simulink model "triangle"  (R2018b)
settings: Solver=FixedStepAuto  StartTime=0.0  StopTime=inf  FixedStep=1/20  RelTol=1e-3  EnableMultiTasking=on
PreLoadFcn:
  | triangle_startup
settings Model: SimulationMode=external  Creator=Josef  LastModifiedBy=Josef
settings SolverCC: PositivePriorityOrder=on
settings OptimizationCC: PassReuseOutputArgsThreshold=0  MaxStackSize=64
settings DebuggingCC: ParameterTunabilityLossMsg=error
settings HardwareCC: ProdBitPerPointer=32  ProdBitPerSizeT=32  ProdBitPerPtrDiffT=32  ProdLargestAtomicInteger=Long  ProdLargestAtomicFloat=Double  ProdWordSize=32  ProdHWDeviceType=ARM Compatible->ARM Cortex  UseEmbeddedCoderFeatures=off
settings SFSimCC: SimUseLocalCustomCode=off  MATLABDynamicMemAlloc=off
settings RTWCC: SystemTargetFile=ert.tlc  HardwareBoard=Raspberry Pi  TLCOptions="-aInlineSetEventsForThisBaseRateFcn=TLC_FALSE -aSuppressMultiTaskScheduler=TLC_FALSE  -aRateBasedStepFcn=0"  TemplateMakefile=ert_default_tmf  GenerateReport=on  RTWUseLocalCustomCode=off  Toolchain=GNU GCC Raspberry Pi  TargetLang=C++
settings CodeAppCC: ForceParamTrailComments=on  OperatorAnnotations=on
settings ERTTargetCC: TargetLangStandard=C++03 (ISO)  ERTCustomFileBanners=off  SupportContinuousTime=on  SupportNonInlinedSFcns=on  RemoveResetFunc=off  SupportVariableSizeSignals=on  ModelStepFunctionPrototypeControlCompliant=off

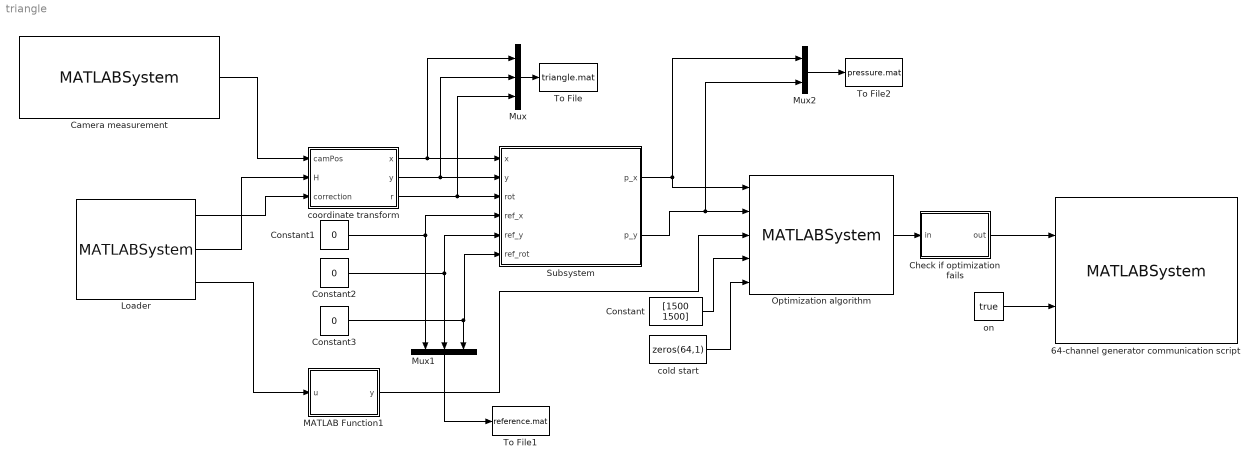
== system triangle ==
  64-channel generator communication script : MATLABSystem  System=NewGenerator  Port=/dev/ttyUSB0  Baud=230400
      mask Type: NewGenerator
      mask Display:
      | disp(['64 phase generator' char(10) ' Port: /dev/ttyUSB0' char(10) ' Baudrate: 230400']);
      | port_label('input',1,'phases');
      | port_label('input',2,'On/Off');
  Camera measurement : MATLABSystem  System=RaspiBallPos  shm_key=3145914  framerate=50  N=1000  objects=1  km=eye( 3 )  notfound=0  execScript=off  concatenateOutputs=off  rotation=on  found_output=off
      mask Type: RaspiBallPos
      mask Display:
      | disp('RaspiBallPos');
      | port_label('output',1,'Position 1 [x;y;r]');
  Check if optimization fails : MATLAB Function  TreatAsAtomicUnit=on
  Constant : Constant  Value=[1500 1500]
  Constant1 : Constant  Value=0
  Constant2 : Constant  Value=0
  Constant3 : Constant  Value=0
  Loader : MATLABSystem  System=Loader  corrFile=correction.bin  H_unFile=H_unrot.bin  heightFile=height.bin
      mask Type: Loader
      mask Display:
      | disp('Loader');
      | port_label('output',1,'correction');
      | port_label('output',2,'H_unrot');
      | port_label('output',3,'height');
  MATLAB Function1 : MATLAB Function  TreatAsAtomicUnit=on
  Mux : Mux  Inputs=3
  Mux1 : Mux  Inputs=3
  Mux2 : Mux  Inputs=2
  Optimization algorithm : MATLABSystem  System=PressurePoints
      mask Type: PressurePoints
      mask Display:
      | disp(['Pressure points' char(10) 'optimization']);
      | port_label('input',1,'x');
      | port_label('input',2,'y');
      | port_label('input',3,'z');
      | port_label('input',4,'Required pressure');
      | port_label('input',5,'Initial condition');
      | port_label('output',1,'Phases');
  Subsystem : Subsystem  mask{triangle_width=0.010, triangle_height=0.013, in_dist=0.0015, out_dist=0.00075}
      mask prompts: triangle_width "Width"; triangle_height "Height"; in_dist "Inner distance"; out_dist "Outer distance"
      mask DialogControl DescGroupVar Prompt: Controller
      mask DialogControl DescTextVar Prompt: Determines position of high-pressure points
      mask DialogControl Container3 Prompt: Triangle
      mask DialogControl Container4 Prompt: Determine pressure points
  To File : ToFile  Filename=triangle.mat  MatrixName=triangle
  To File1 : ToFile  Filename=reference.mat  MatrixName=reference
  To File2 : ToFile  Filename=pressure.mat  MatrixName=pressure
  cold start : Constant  Value=zeros(64,1)
  coordinate transform : MATLAB Function  TreatAsAtomicUnit=on
  on : Constant  Value=true
  wires:
  Camera measurement/1 -> coordinate transform/1(camPos)
  Optimization algorithm/1 -> Check if optimization fails/1(in)
  cold start/1 -> Optimization algorithm/5
  on/1 -> 64-channel generator communication script/2
  Check if optimization fails/1(out) -> 64-channel generator communication script/1
  Loader/1 -> coordinate transform/3(correction)
  Loader/2 -> coordinate transform/2(H)
  Loader/3 -> MATLAB Function1/1(u)
  MATLAB Function1/1(y) -> Optimization algorithm/3
  Constant/1 -> Optimization algorithm/4
  coordinate transform/1(x) -> Mux/1, Subsystem/1(x)
  coordinate transform/2(y) -> Mux/2, Subsystem/2(y)
  coordinate transform/3(r) -> Mux/3, Subsystem/3(rot)
  Constant1/1 -> Subsystem/4(ref_x), Mux1/1
  Constant2/1 -> Subsystem/5(ref_y), Mux1/2
  Constant3/1 -> Subsystem/6(ref_rot), Mux1/3
  Subsystem/1(p_x) -> Mux2/1, Optimization algorithm/1
  Subsystem/2(p_y) -> Mux2/2, Optimization algorithm/2
  Mux/1 -> To File/1
  Mux1/1 -> To File1/1
  Mux2/1 -> To File2/1

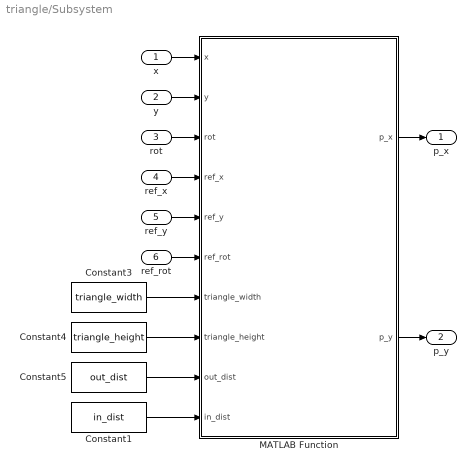
== system triangle/Subsystem ==
  x : Inport
  y : Inport  Port=2
  rot : Inport  Port=3
  ref_x : Inport  Port=4
  ref_y : Inport  Port=5
  ref_rot : Inport  Port=6
  Constant1 : Constant  Value=in_dist
  Constant3 : Constant  Value=triangle_width
  Constant4 : Constant  Value=triangle_height
  Constant5 : Constant  Value=out_dist
  MATLAB Function : MATLAB Function  TreatAsAtomicUnit=on
  p_x : Outport
  p_y : Outport  Port=2
  wires:
  MATLAB Function/1(p_x) -> p_x/1
  rot/1 -> MATLAB Function/3(rot)
  Constant3/1 -> MATLAB Function/7(triangle_width)
  x/1 -> MATLAB Function/1(x)
  ref_x/1 -> MATLAB Function/4(ref_x)
  Constant4/1 -> MATLAB Function/8(triangle_height)
  y/1 -> MATLAB Function/2(y)
  Constant5/1 -> MATLAB Function/9(out_dist)
  ref_y/1 -> MATLAB Function/5(ref_y)
  ref_rot/1 -> MATLAB Function/6(ref_rot)
  MATLAB Function/2(p_y) -> p_y/1
  Constant1/1 -> MATLAB Function/10(in_dist)

== matlab function triangle/coordinate transform ==
  data: x output; camPos input; y output; H input; correction input; r output
function [x,y,r] = trans(camPos, H, correction)
    [x,y] = coordTransform(H, camPos(1:2), correction);
    r = camPos(3);
end

== matlab function triangle/Subsystem/MATLAB Function ==
  data: x input; p_x output; y input; rot input; ref_x input; ref_y input; ref_rot input; triangle_width input; triangle_height input; p_y output; out_dist input; in_dist input
function [p_x, p_y] = determine_pressure_points(x, y, rot, ref_x, ref_y, ref_rot, triangle_width, triangle_height, out_dist, in_dist)
    rot_mat = [cos(rot), -sin(rot); sin(rot), cos(rot)];
    ref_rot_mat = [cos(ref_rot), -sin(ref_rot); sin(ref_rot), cos(ref_rot)];
    T = [x;y];
    P = [ref_x;ref_y];
    
    dx = triangle_height/3 + out_dist;
    dy = triangle_width/2 + out_dist;   
    dxr = triangle_height/3 - in_dist;
    dyr = triangle_width/2 - in_dist;
    TA = rot_mat * [-dxr;dyr];
    TB = rot_mat * [-dxr;-dyr];
    TC = rot_mat * [2*dxr;0];
    TP = P - T;
    A = T + TA;
    B = T + TB;
    C = T + TC;
    
    total_dist = in_dist + out_dist;
	AA_ref = - TA + TP + ref_rot_mat * [-dx;dy];
    if norm(AA_ref) > total_dist
        AA_ref = AA_ref / norm(AA_ref) * (total_dist);
    end
	BB_ref = - TB + TP +  ref_rot_mat * [-dx;-dy];
    if norm(BB_ref) > total_dist
        BB_ref = BB_ref / norm(BB_ref) * (total_dist);
    end
	CC_ref = - TC + TP +  ref_rot_mat * [2*dx;0];
    if norm(CC_ref) > total_dist
        CC_ref = CC_ref / norm(CC_ref) * (total_dist);
    end
    
    points = [A + AA_ref,B + BB_ref,C + CC_ref];
    
    [~, indices] = sort([AA_ref'*TP, BB_ref'*TP, CC_ref'*TP]);
    p_x = points(1,indices(2:3));
    p_y = points(2,indices(2:3));

== matlab function triangle/Check if optimization fails ==
  data: in input; out output
function out = NaNcontrol(in)
    if isnan(in)
        out = zeros(64,1);
    else
        out = in;
    end
% % end

== matlab function triangle/MATLAB Function1 ==
  data: u input; y output
function y = duplicate(u)

y = [u, u];
